simulink model "nonlinear_model"  (R2017b)
settings: Solver=VariableStepAuto  StartTime=0.0  StopTime=5  RelTol=1e-3
values from neighbouring files (symbols this model uses):
  altitude = input('Enter the altitude for the simulation (ft)  :  ')    [FindF16Dynamics.m]    (also in run_me.m = input(' altitude ( 0 ~ 40000 ft ) : '); trim_F16.m = alt)
  control_trim = u0    [find_trim.m]
  state_trim = steady_state( state )    [find_trim.m]
  velocity = input('Enter the velocity for the simulation (ft/s):  ')    [FindF16Dynamics.m]    (also in run_me.m = input(' true velocity ( 350 ~ 1000 ft/sec ) : '); trim_F16.m = vel)
libraries: simulink x7
settings Model: Creator=monster  LastModifiedBy=monster

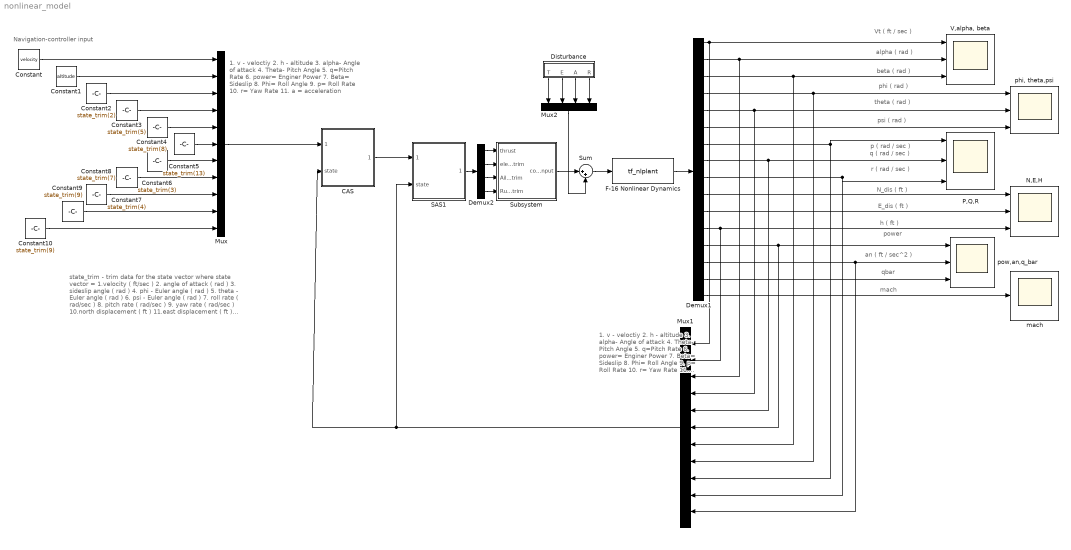
== system nonlinear_model ==
  note: state_trim   - trim data for the state vector where
      |       state vector =
      | 1.velocity             ( ft/sec )
      | 2. angle of attack      ( rad )
      |  3. sideslip angle       ( rad )
      | 4. phi   - Euler angle  ( rad )
      | 5. theta - Euler angle  ( rad )
      |    6. psi   - Euler angle  ( rad )
      |   7. roll rate            ( rad/sec )
      | 8. pitch rate           ( rad/sec )
      |  9. yaw rate             ( rad/sec )
      | 10.north displacement   ( ft )
      | 11.east displacement    ( ft )
      | 12.altitude             ( ft )
      | 13.power  ( percent, 0 <= pow <= 100 )
  note: phi ( rad )
  note: theta ( rad )
  note: h ( ft )
  note: E_dis ( ft )
  note: power
  note: an ( ft / sec^2 )
  note: mach
  note: Vt ( ft / sec )
  note: p ( rad / sec )
  note: r ( rad / sec )
  note: q ( rad / sec )
  note: N_dis ( ft )
  note: qbar
  note: alpha ( rad )
  note: beta ( rad )
  note: psi ( rad )
  note: 1. v - veloctiy
      |
      | 2. h - altitude
      |
      | 3. alpha- Angle of attack
      |
      | 4. Theta- Pitch Angle
      |
      | 5. q=Pitch Rate
      |
      | 6. power= Enginer Power
      |
      | 7. Beta= Sideslip
      |
      | 8. Phi= Roll Angle
      |
      | 9. p= Roll Rate
      |
      | 10. r= Yaw Rate
      |
      | 11. a = acceleration
  note: 1. v - veloctiy
      |
      | 2. h - altitude
      |
      | 3. alpha- Angle of attack
      |
      | 4. Theta- Pitch Angle
      |
      | 5. q=Pitch Rate
      |
      | 6. power= Enginer Power
      |
      | 7. Beta= Sideslip
      |
      | 8. Phi= Roll Angle
      |
      | 9. p= Roll Rate
      |
      | 10. r= Yaw Rate
      |
      | 11. a= acceleration
  note: Navigation-controller input
  " Disturbance" : Subsystem
  CAS : Subsystem
  Constant : Constant  Value=velocity
  Constant1 : Constant  Value=altitude
  Constant10 : Constant  Value=state_trim(9)
  Constant2 : Constant  Value=state_trim(2)
  Constant3 : Constant  Value=state_trim(5)
  Constant4 : Constant  Value=state_trim(8)
  Constant5 : Constant  Value=state_trim(13)
  Constant6 : Constant  Value=state_trim(3)
  Constant7 : Constant  Value=state_trim(4)
  Constant8 : Constant  Value=state_trim(7)
  Constant9 : Constant  Value=state_trim(9)
  Demux1 : Demux  Outputs=16
  Demux2 : Demux
  F-16 Nonlinear Dynamics : S-Function  FunctionName=tf_nlplant  Parameters="state_trim,  xcg"  SFunctionDeploymentMode=off  EnableBusSupport=off
  Mux : Mux  Inputs=11
  Mux1 : Mux  Inputs=11
  Mux2 : Mux
  N,E,H : Scope  NumInputPorts=3
  P,Q,R : Scope  NumInputPorts=3
  SAS1 : Subsystem
  Subsystem : Subsystem
  Sum : Sum  Inputs=|++
  "V,alpha, beta" : Scope  NumInputPorts=3
  mach : Scope
  "phi, theta,psi" : Scope  NumInputPorts=3
  pow,an,q_bar : Scope  NumInputPorts=3
  wires:
  Demux1/11 -> N,E,H/2
  Demux1/12 -> N,E,H/3, Mux1/2
  Demux1/1 -> Mux1/1, "V,alpha, beta"/1
  Demux1/15 -> pow,an,q_bar/3
  Demux1/2 -> "V,alpha, beta"/2, Mux1/3
  Demux1/4 -> Mux1/8, "phi, theta,psi"/1
  Demux1/9 -> Mux1/10, P,Q,R/3
  Demux1/8 -> Mux1/5, P,Q,R/2
  Demux1/10 -> N,E,H/1
  Demux1/5 -> Mux1/4, "phi, theta,psi"/2
  Demux1/3 -> Mux1/7, "V,alpha, beta"/3
  Demux1/7 -> Mux1/9, P,Q,R/1
  Demux1/6 -> "phi, theta,psi"/3
  Demux1/16 -> mach/1
  Demux1/13 -> Mux1/6, pow,an,q_bar/1
  " Disturbance"/3(A) -> Mux2/3
  " Disturbance"/2(E) -> Mux2/2
  Constant/1 -> Mux/1
  Constant9/1 -> Mux/10
  Constant6/1 -> Mux/7
  Constant2/1 -> Mux/3
  Constant1/1 -> Mux/2
  Constant4/1 -> Mux/5
  " Disturbance"/1(T) -> Mux2/1
  Constant7/1 -> Mux/8
  Constant8/1 -> Mux/9
  Constant3/1 -> Mux/4
  Demux2/4 -> Subsystem/4(Rudder_trim)
  Demux2/1 -> Subsystem/1(thrust)
  Demux2/2 -> Subsystem/2(elevator_trim)
  Subsystem/1(control_input) -> Sum/1
  Mux/1 -> CAS/1(reference)
  Constant10/1 -> Mux/11
  Constant5/1 -> Mux/6
  Sum/1 -> F-16 Nonlinear Dynamics/1
  Demux2/3 -> Subsystem/3(Aileron_trim)
  Mux2/1 -> Sum/2
  " Disturbance"/4(R) -> Mux2/4
  SAS1/1(control_input) -> Demux2/1
  F-16 Nonlinear Dynamics/1 -> Demux1/1
  Demux1/14 -> Mux1/11, pow,an,q_bar/2
  Mux1/1 -> SAS1/2(state), CAS/2(state)
  CAS/1(control_input) -> SAS1/1(reference)

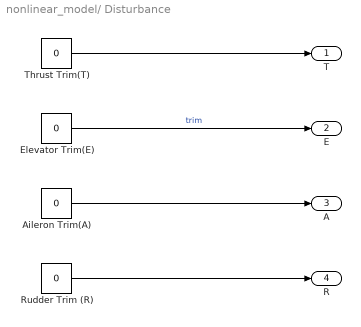
== system nonlinear_model/ Disturbance ==
  "Aileron Trim(A) " : Constant  Value=0
  "Elevator Trim(E) " : Constant  Value=0  VectorParams1D=off
  Rudder Trim (R) : Constant  Value=0
  "Thrust Trim(T) " : Constant  Value=0
  T : Outport
  E : Outport  Port=2
  A : Outport  Port=3
  R : Outport  Port=4
  wires:
  "Aileron Trim(A) "/1 -> A/1
  "Elevator Trim(E) "/1 -> E/1  "trim"
  "Thrust Trim(T) "/1 -> T/1
  Rudder Trim (R)/1 -> R/1

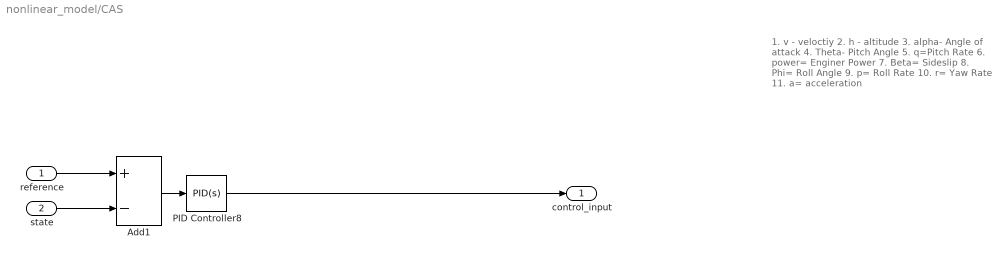
== system nonlinear_model/CAS ==
  note: 1. v - veloctiy
      |
      | 2. h - altitude
      |
      | 3. alpha- Angle of attack
      |
      | 4. Theta- Pitch Angle
      |
      | 5. q=Pitch Rate
      |
      | 6. power= Enginer Power
      |
      | 7. Beta= Sideslip
      |
      | 8. Phi= Roll Angle
      |
      | 9. p= Roll Rate
      |
      | 10. r= Yaw Rate
      |
      | 11. a= acceleration
  reference : Inport
  state : Inport  Port=2
  Add1 : Sum  Inputs=+-
  PID Controller8 : simulink/Continuous/PID Controller  Controller=PID  TimeDomain=Continuous-time  SampleTime=-1  IntegratorMethod=Forward Euler  FilterMethod=Forward Euler  Form=Parallel  UseFilter=on  ControllerParametersSource=internal  P=-49327.5398646116  I=-459229.123376859  D=-1288.80480278299  N=1181.77739704053  InitialConditionSource=internal  InitialConditionForIntegrator=0  InitialConditionForFilter=0  ExternalReset=none  LimitOutput=off  UpperSaturationLimit=inf  LowerSaturationLimit=-inf  LinearizeAsGain=on  AntiWindupMode=none  Kb=1  TrackingMode=off  Kt=1  PParamMin=[]  PParamMax=[]  IParamMin=[]  IParamMax=[]  DParamMin=[]  DParamMax=[]  NParamMin=[]  NParamMax=[]  KbParamMin=[]  KbParamMax=[]  KtParamMin=[]  KtParamMax=[]  POutMin=[]  POutMax=[]  IOutMin=[]  IOutMax=[]  DOutMin=[]  DOutMax=[]  NOutMin=[]  NOutMax=[]  KbOutMin=[]  KbOutMax=[]  KtOutMin=[]  KtOutMax=[]  IntegratorOutMin=[]  IntegratorOutMax=[]  FilterOutMin=[]  FilterOutMax=[]  SumOutMin=[]  SumOutMax=[]  SumI1OutMin=[]  SumI1OutMax=[]  SumI2OutMin=[]  SumI2OutMax=[]  SumI3OutMin=[]  SumI3OutMax=[]  SumDOutMin=[]  SumDOutMax=[]  SaturationOutMin=[]  SaturationOutMax=[]  IntegratorContinuousStateAttributes=''  IntegratorStateMustResolveToSignalObject=off  IntegratorRTWStateStorageClass=Auto  FilterContinuousStateAttributes=''  FilterStateMustResolveToSignalObject=off  FilterRTWStateStorageClass=Auto  DifferentiatorICPrevScaledInput=0  DifferentiatorOutMin=[]  DifferentiatorOutMax=[]  InitialConditionSetting=State (most efficient)  FilterDiffOutCoefMin=[]  FilterDiffOutCoefMax=[]  SumDenOutMin=[]  SumDenOutMax=[]  SumNumOutMin=[]  SumNumOutMax=[]  ReciprocalOutMin=[]  ReciprocalOutMax=[]  DivideOutMin=[]  DivideOutMax=[]  TunerSelectOption=Transfer Function Based (PID Tuner App)
  control_input : Outport
  wires:
  PID Controller8/1 -> control_input/1
  Add1/1 -> PID Controller8/1
  reference/1 -> Add1/1
  state/1 -> Add1/2

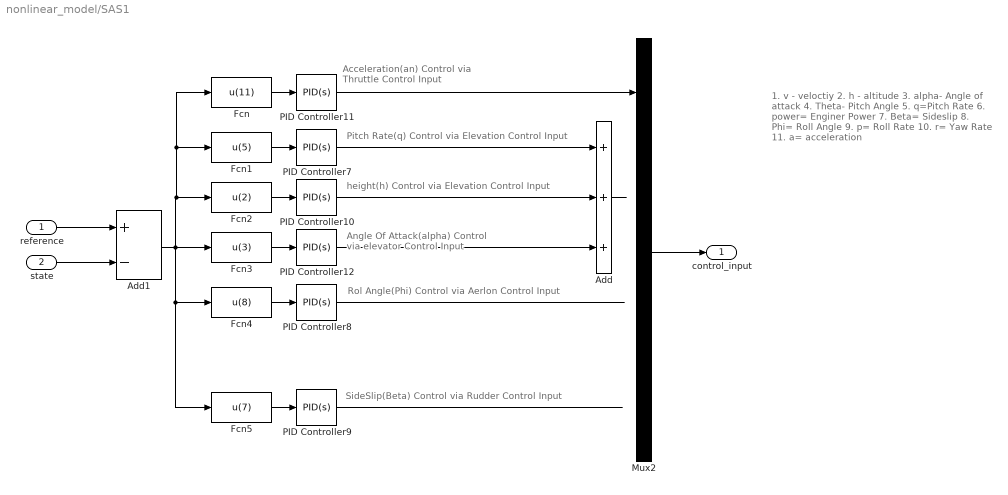
== system nonlinear_model/SAS1 ==
  note: Rol Angle(Phi) Control via Aerlon Control Input
  note: height(h) Control via Elevation Control Input
  note: Pitch Rate(q) Control via Elevation Control Input
  note: Acceleration(an) Control via Thruttle Control Input
  note: Angle Of Attack(alpha) Control via elevator Control Input
  note: SideSlip(Beta) Control via Rudder Control Input
  note: 1. v - veloctiy
      |
      | 2. h - altitude
      |
      | 3. alpha- Angle of attack
      |
      | 4. Theta- Pitch Angle
      |
      | 5. q=Pitch Rate
      |
      | 6. power= Enginer Power
      |
      | 7. Beta= Sideslip
      |
      | 8. Phi= Roll Angle
      |
      | 9. p= Roll Rate
      |
      | 10. r= Yaw Rate
      |
      | 11. a= acceleration
  reference : Inport
  state : Inport  Port=2
  Add : Sum  Inputs=+++
  Add1 : Sum  Inputs=+-
  Fcn : Fcn  Expr=u(11)
  Fcn1 : Fcn  Expr=u(5)
  Fcn2 : Fcn  Expr=u(2)
  Fcn3 : Fcn  Expr=u(3)
  Fcn4 : Fcn  Expr=u(8)
  Fcn5 : Fcn  Expr=u(7)
  Mux2 : Mux
  PID Controller10 : simulink/Continuous/PID Controller  Controller=PID  TimeDomain=Continuous-time  SampleTime=-1  IntegratorMethod=Forward Euler  FilterMethod=Forward Euler  Form=Parallel  UseFilter=on  ControllerParametersSource=internal  P=24508600.1259152  I=4501969741.89748  D=28958.3047379278  N=690409.793644926  InitialConditionSource=internal  InitialConditionForIntegrator=0  InitialConditionForFilter=0  ExternalReset=none  LimitOutput=off  UpperSaturationLimit=inf  LowerSaturationLimit=-inf  LinearizeAsGain=on  AntiWindupMode=none  Kb=1  TrackingMode=off  Kt=1  PParamMin=[]  PParamMax=[]  IParamMin=[]  IParamMax=[]  DParamMin=[]  DParamMax=[]  NParamMin=[]  NParamMax=[]  KbParamMin=[]  KbParamMax=[]  KtParamMin=[]  KtParamMax=[]  POutMin=[]  POutMax=[]  IOutMin=[]  IOutMax=[]  DOutMin=[]  DOutMax=[]  NOutMin=[]  NOutMax=[]  KbOutMin=[]  KbOutMax=[]  KtOutMin=[]  KtOutMax=[]  IntegratorOutMin=[]  IntegratorOutMax=[]  FilterOutMin=[]  FilterOutMax=[]  SumOutMin=[]  SumOutMax=[]  SumI1OutMin=[]  SumI1OutMax=[]  SumI2OutMin=[]  SumI2OutMax=[]  SumI3OutMin=[]  SumI3OutMax=[]  SumDOutMin=[]  SumDOutMax=[]  SaturationOutMin=[]  SaturationOutMax=[]  IntegratorContinuousStateAttributes=''  IntegratorStateMustResolveToSignalObject=off  IntegratorRTWStateStorageClass=Auto  FilterContinuousStateAttributes=''  FilterStateMustResolveToSignalObject=off  FilterRTWStateStorageClass=Auto  DifferentiatorICPrevScaledInput=0  DifferentiatorOutMin=[]  DifferentiatorOutMax=[]  InitialConditionSetting=State (most efficient)  FilterDiffOutCoefMin=[]  FilterDiffOutCoefMax=[]  SumDenOutMin=[]  SumDenOutMax=[]  SumNumOutMin=[]  SumNumOutMax=[]  ReciprocalOutMin=[]  ReciprocalOutMax=[]  DivideOutMin=[]  DivideOutMax=[]  TunerSelectOption=Transfer Function Based (PID Tuner App)
  PID Controller11 : simulink/Continuous/PID Controller  Controller=PID  TimeDomain=Continuous-time  SampleTime=-1  IntegratorMethod=Forward Euler  FilterMethod=Forward Euler  Form=Parallel  UseFilter=on  ControllerParametersSource=internal  P=13329483.1324469  I=392847306.175743  D=98980.5300334758  N=109037.560099343  InitialConditionSource=internal  InitialConditionForIntegrator=0  InitialConditionForFilter=0  ExternalReset=none  LimitOutput=off  UpperSaturationLimit=inf  LowerSaturationLimit=-inf  LinearizeAsGain=on  AntiWindupMode=none  Kb=1  TrackingMode=off  Kt=1  PParamMin=[]  PParamMax=[]  IParamMin=[]  IParamMax=[]  DParamMin=[]  DParamMax=[]  NParamMin=[]  NParamMax=[]  KbParamMin=[]  KbParamMax=[]  KtParamMin=[]  KtParamMax=[]  POutMin=[]  POutMax=[]  IOutMin=[]  IOutMax=[]  DOutMin=[]  DOutMax=[]  NOutMin=[]  NOutMax=[]  KbOutMin=[]  KbOutMax=[]  KtOutMin=[]  KtOutMax=[]  IntegratorOutMin=[]  IntegratorOutMax=[]  FilterOutMin=[]  FilterOutMax=[]  SumOutMin=[]  SumOutMax=[]  SumI1OutMin=[]  SumI1OutMax=[]  SumI2OutMin=[]  SumI2OutMax=[]  SumI3OutMin=[]  SumI3OutMax=[]  SumDOutMin=[]  SumDOutMax=[]  SaturationOutMin=[]  SaturationOutMax=[]  IntegratorContinuousStateAttributes=''  IntegratorStateMustResolveToSignalObject=off  IntegratorRTWStateStorageClass=Auto  FilterContinuousStateAttributes=''  FilterStateMustResolveToSignalObject=off  FilterRTWStateStorageClass=Auto  DifferentiatorICPrevScaledInput=0  DifferentiatorOutMin=[]  DifferentiatorOutMax=[]  InitialConditionSetting=State (most efficient)  FilterDiffOutCoefMin=[]  FilterDiffOutCoefMax=[]  SumDenOutMin=[]  SumDenOutMax=[]  SumNumOutMin=[]  SumNumOutMax=[]  ReciprocalOutMin=[]  ReciprocalOutMax=[]  DivideOutMin=[]  DivideOutMax=[]  TunerSelectOption=Transfer Function Based (PID Tuner App)
  PID Controller12 : simulink/Continuous/PID Controller  Controller=PID  TimeDomain=Continuous-time  SampleTime=-1  IntegratorMethod=Forward Euler  FilterMethod=Forward Euler  Form=Parallel  UseFilter=on  ControllerParametersSource=internal  P=-170.14183467408  I=-465.695324804371  D=-13.6839697818054  N=105.697856042613  InitialConditionSource=internal  InitialConditionForIntegrator=0  InitialConditionForFilter=0  ExternalReset=none  LimitOutput=off  UpperSaturationLimit=inf  LowerSaturationLimit=-inf  LinearizeAsGain=on  AntiWindupMode=none  Kb=1  TrackingMode=off  Kt=1  PParamMin=[]  PParamMax=[]  IParamMin=[]  IParamMax=[]  DParamMin=[]  DParamMax=[]  NParamMin=[]  NParamMax=[]  KbParamMin=[]  KbParamMax=[]  KtParamMin=[]  KtParamMax=[]  POutMin=[]  POutMax=[]  IOutMin=[]  IOutMax=[]  DOutMin=[]  DOutMax=[]  NOutMin=[]  NOutMax=[]  KbOutMin=[]  KbOutMax=[]  KtOutMin=[]  KtOutMax=[]  IntegratorOutMin=[]  IntegratorOutMax=[]  FilterOutMin=[]  FilterOutMax=[]  SumOutMin=[]  SumOutMax=[]  SumI1OutMin=[]  SumI1OutMax=[]  SumI2OutMin=[]  SumI2OutMax=[]  SumI3OutMin=[]  SumI3OutMax=[]  SumDOutMin=[]  SumDOutMax=[]  SaturationOutMin=[]  SaturationOutMax=[]  IntegratorContinuousStateAttributes=''  IntegratorStateMustResolveToSignalObject=off  IntegratorRTWStateStorageClass=Auto  FilterContinuousStateAttributes=''  FilterStateMustResolveToSignalObject=off  FilterRTWStateStorageClass=Auto  DifferentiatorICPrevScaledInput=0  DifferentiatorOutMin=[]  DifferentiatorOutMax=[]  InitialConditionSetting=State (most efficient)  FilterDiffOutCoefMin=[]  FilterDiffOutCoefMax=[]  SumDenOutMin=[]  SumDenOutMax=[]  SumNumOutMin=[]  SumNumOutMax=[]  ReciprocalOutMin=[]  ReciprocalOutMax=[]  DivideOutMin=[]  DivideOutMax=[]  TunerSelectOption=Transfer Function Based (PID Tuner App)
  PID Controller7 : simulink/Continuous/PID Controller  Controller=PID  TimeDomain=Continuous-time  SampleTime=-1  IntegratorMethod=Forward Euler  FilterMethod=Forward Euler  Form=Parallel  UseFilter=on  ControllerParametersSource=internal  P=-2409.99420452658  I=-41171.6281036838  D=-4.63151383685818  N=352.425457454863  InitialConditionSource=internal  InitialConditionForIntegrator=0  InitialConditionForFilter=0  ExternalReset=none  LimitOutput=off  UpperSaturationLimit=inf  LowerSaturationLimit=-inf  LinearizeAsGain=on  AntiWindupMode=none  Kb=1  TrackingMode=off  Kt=1  PParamMin=[]  PParamMax=[]  IParamMin=[]  IParamMax=[]  DParamMin=[]  DParamMax=[]  NParamMin=[]  NParamMax=[]  KbParamMin=[]  KbParamMax=[]  KtParamMin=[]  KtParamMax=[]  POutMin=[]  POutMax=[]  IOutMin=[]  IOutMax=[]  DOutMin=[]  DOutMax=[]  NOutMin=[]  NOutMax=[]  KbOutMin=[]  KbOutMax=[]  KtOutMin=[]  KtOutMax=[]  IntegratorOutMin=[]  IntegratorOutMax=[]  FilterOutMin=[]  FilterOutMax=[]  SumOutMin=[]  SumOutMax=[]  SumI1OutMin=[]  SumI1OutMax=[]  SumI2OutMin=[]  SumI2OutMax=[]  SumI3OutMin=[]  SumI3OutMax=[]  SumDOutMin=[]  SumDOutMax=[]  SaturationOutMin=[]  SaturationOutMax=[]  IntegratorContinuousStateAttributes=''  IntegratorStateMustResolveToSignalObject=off  IntegratorRTWStateStorageClass=Auto  FilterContinuousStateAttributes=''  FilterStateMustResolveToSignalObject=off  FilterRTWStateStorageClass=Auto  DifferentiatorICPrevScaledInput=0  DifferentiatorOutMin=[]  DifferentiatorOutMax=[]  InitialConditionSetting=State (most efficient)  FilterDiffOutCoefMin=[]  FilterDiffOutCoefMax=[]  SumDenOutMin=[]  SumDenOutMax=[]  SumNumOutMin=[]  SumNumOutMax=[]  ReciprocalOutMin=[]  ReciprocalOutMax=[]  DivideOutMin=[]  DivideOutMax=[]  TunerSelectOption=Transfer Function Based (PID Tuner App)
  PID Controller8 : simulink/Continuous/PID Controller  Controller=PID  TimeDomain=Continuous-time  SampleTime=-1  IntegratorMethod=Forward Euler  FilterMethod=Forward Euler  Form=Parallel  UseFilter=on  ControllerParametersSource=internal  P=-49327.5398646116  I=-459229.123376859  D=-1288.80480278299  N=1181.77739704053  InitialConditionSource=internal  InitialConditionForIntegrator=0  InitialConditionForFilter=0  ExternalReset=none  LimitOutput=off  UpperSaturationLimit=inf  LowerSaturationLimit=-inf  LinearizeAsGain=on  AntiWindupMode=none  Kb=1  TrackingMode=off  Kt=1  PParamMin=[]  PParamMax=[]  IParamMin=[]  IParamMax=[]  DParamMin=[]  DParamMax=[]  NParamMin=[]  NParamMax=[]  KbParamMin=[]  KbParamMax=[]  KtParamMin=[]  KtParamMax=[]  POutMin=[]  POutMax=[]  IOutMin=[]  IOutMax=[]  DOutMin=[]  DOutMax=[]  NOutMin=[]  NOutMax=[]  KbOutMin=[]  KbOutMax=[]  KtOutMin=[]  KtOutMax=[]  IntegratorOutMin=[]  IntegratorOutMax=[]  FilterOutMin=[]  FilterOutMax=[]  SumOutMin=[]  SumOutMax=[]  SumI1OutMin=[]  SumI1OutMax=[]  SumI2OutMin=[]  SumI2OutMax=[]  SumI3OutMin=[]  SumI3OutMax=[]  SumDOutMin=[]  SumDOutMax=[]  SaturationOutMin=[]  SaturationOutMax=[]  IntegratorContinuousStateAttributes=''  IntegratorStateMustResolveToSignalObject=off  IntegratorRTWStateStorageClass=Auto  FilterContinuousStateAttributes=''  FilterStateMustResolveToSignalObject=off  FilterRTWStateStorageClass=Auto  DifferentiatorICPrevScaledInput=0  DifferentiatorOutMin=[]  DifferentiatorOutMax=[]  InitialConditionSetting=State (most efficient)  FilterDiffOutCoefMin=[]  FilterDiffOutCoefMax=[]  SumDenOutMin=[]  SumDenOutMax=[]  SumNumOutMin=[]  SumNumOutMax=[]  ReciprocalOutMin=[]  ReciprocalOutMax=[]  DivideOutMin=[]  DivideOutMax=[]  TunerSelectOption=Transfer Function Based (PID Tuner App)
  PID Controller9 : simulink/Continuous/PID Controller  Controller=PID  TimeDomain=Continuous-time  SampleTime=-1  IntegratorMethod=Forward Euler  FilterMethod=Forward Euler  Form=Parallel  UseFilter=on  ControllerParametersSource=internal  P=908.491475757153  I=143.160579860217  D=1280.97081759687  N=3086.89831654681  InitialConditionSource=internal  InitialConditionForIntegrator=0  InitialConditionForFilter=0  ExternalReset=none  LimitOutput=off  UpperSaturationLimit=inf  LowerSaturationLimit=-inf  LinearizeAsGain=on  AntiWindupMode=none  Kb=1  TrackingMode=off  Kt=1  PParamMin=[]  PParamMax=[]  IParamMin=[]  IParamMax=[]  DParamMin=[]  DParamMax=[]  NParamMin=[]  NParamMax=[]  KbParamMin=[]  KbParamMax=[]  KtParamMin=[]  KtParamMax=[]  POutMin=[]  POutMax=[]  IOutMin=[]  IOutMax=[]  DOutMin=[]  DOutMax=[]  NOutMin=[]  NOutMax=[]  KbOutMin=[]  KbOutMax=[]  KtOutMin=[]  KtOutMax=[]  IntegratorOutMin=[]  IntegratorOutMax=[]  FilterOutMin=[]  FilterOutMax=[]  SumOutMin=[]  SumOutMax=[]  SumI1OutMin=[]  SumI1OutMax=[]  SumI2OutMin=[]  SumI2OutMax=[]  SumI3OutMin=[]  SumI3OutMax=[]  SumDOutMin=[]  SumDOutMax=[]  SaturationOutMin=[]  SaturationOutMax=[]  IntegratorContinuousStateAttributes=''  IntegratorStateMustResolveToSignalObject=off  IntegratorRTWStateStorageClass=Auto  FilterContinuousStateAttributes=''  FilterStateMustResolveToSignalObject=off  FilterRTWStateStorageClass=Auto  DifferentiatorICPrevScaledInput=0  DifferentiatorOutMin=[]  DifferentiatorOutMax=[]  InitialConditionSetting=State (most efficient)  FilterDiffOutCoefMin=[]  FilterDiffOutCoefMax=[]  SumDenOutMin=[]  SumDenOutMax=[]  SumNumOutMin=[]  SumNumOutMax=[]  ReciprocalOutMin=[]  ReciprocalOutMax=[]  DivideOutMin=[]  DivideOutMax=[]  TunerSelectOption=Transfer Function Based (PID Tuner App)
  control_input : Outport
  wires:
  Mux2/1 -> control_input/1
  PID Controller11/1 -> Mux2/1
  Fcn5/1 -> PID Controller9/1
  Fcn3/1 -> PID Controller12/1
  PID Controller7/1 -> Add/1
  Fcn2/1 -> PID Controller10/1
  Fcn1/1 -> PID Controller7/1
  PID Controller8/1 -> ?
  Fcn4/1 -> PID Controller8/1
  Fcn/1 -> PID Controller11/1
  PID Controller10/1 -> Add/2
  Add/1 -> ?
  PID Controller12/1 -> Add/3
  PID Controller9/1 -> ?
  reference/1 -> Add1/1
  state/1 -> Add1/2
  Add1/1 -> Fcn2/1, Fcn1/1, Fcn/1, Fcn5/1, Fcn4/1, Fcn3/1

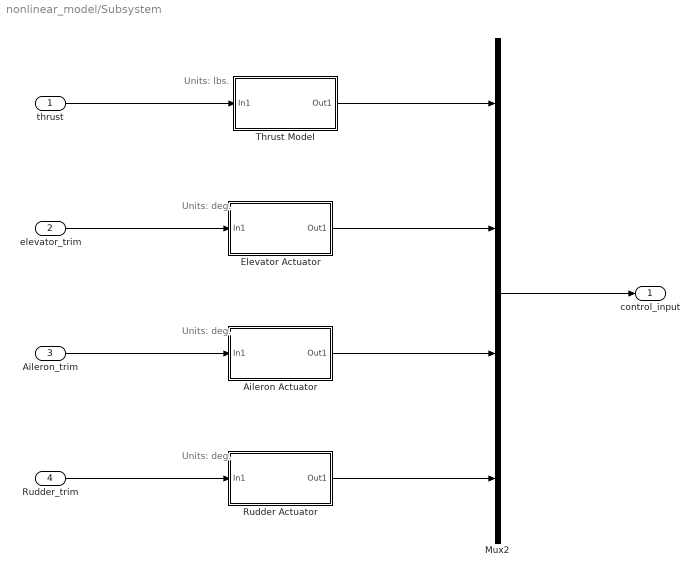
== system nonlinear_model/Subsystem ==
  note: Units: deg.
  note: Units: deg.
  note: Units: lbs.
  note: Units: deg.
  thrust : Inport
  elevator_trim : Inport  Port=2
  Aileron_trim : Inport  Port=3
  Rudder_trim : Inport  Port=4
  Aileron Actuator : Subsystem  AncestorBlock=F16_Actuator_Library/Aileron Actuator
  Elevator Actuator : Subsystem  AncestorBlock=F16_Actuator_Library/Elevator Actuator
  Mux2 : Mux
  Rudder Actuator : Subsystem  AncestorBlock=F16_Actuator_Library/Rudder Actuator
  Thrust Model : Subsystem  AncestorBlock=F16_Actuator_Library/Thrust Model
  control_input : Outport
  wires:
  thrust/1 -> Thrust Model/1(In1)
  Aileron Actuator/1(Out1) -> Mux2/3
  Rudder_trim/1 -> Rudder Actuator/1(In1)
  Elevator Actuator/1(Out1) -> Mux2/2
  Rudder Actuator/1(Out1) -> Mux2/4
  elevator_trim/1 -> Elevator Actuator/1(In1)
  Aileron_trim/1 -> Aileron Actuator/1(In1)
  Thrust Model/1(Out1) -> Mux2/1
  Mux2/1 -> control_input/1

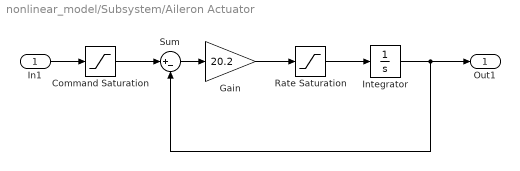
== system nonlinear_model/Subsystem/Aileron Actuator ==
  In1 : Inport
  Command Saturation : Saturate  UpperLimit=21.5  LowerLimit=-21.5
  Gain : Gain  Gain=20.2  SaturateOnIntegerOverflow=on  OutDataTypeStr=Inherit: Same as input  ParamDataTypeStr=Inherit: Same as input
  "Integrator " : Integrator  InitialCondition=control_trim(2)  UpperSaturationLimit=21.5  LowerSaturationLimit=-21.5
  Rate Saturation : Saturate  UpperLimit=80  LowerLimit=-80
  Sum : Sum  Inputs=|+-  SaturateOnIntegerOverflow=on  InputSameDT=on  OutDataTypeStr=Inherit: Same as first input
  Out1 : Outport
  wires:
  "Integrator "/1 -> Sum/2, Out1/1
  Rate Saturation/1 -> "Integrator "/1
  Gain/1 -> Rate Saturation/1
  Sum/1 -> Gain/1
  Command Saturation/1 -> Sum/1
  In1/1 -> Command Saturation/1

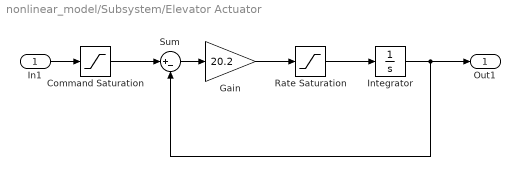
== system nonlinear_model/Subsystem/Elevator Actuator ==
  In1 : Inport
  Command Saturation : Saturate  UpperLimit=25  LowerLimit=-25
  Gain : Gain  Gain=20.2  SaturateOnIntegerOverflow=on  OutDataTypeStr=Inherit: Same as input  ParamDataTypeStr=Inherit: Same as input
  "Integrator " : Integrator  InitialCondition=control_trim(2)  UpperSaturationLimit=25  LowerSaturationLimit=-25
  Rate Saturation : Saturate  UpperLimit=60  LowerLimit=-60
  Sum : Sum  Inputs=|+-  SaturateOnIntegerOverflow=on  InputSameDT=on  OutDataTypeStr=Inherit: Same as first input
  Out1 : Outport
  wires:
  "Integrator "/1 -> Sum/2, Out1/1
  Rate Saturation/1 -> "Integrator "/1
  Gain/1 -> Rate Saturation/1
  Sum/1 -> Gain/1
  Command Saturation/1 -> Sum/1
  In1/1 -> Command Saturation/1

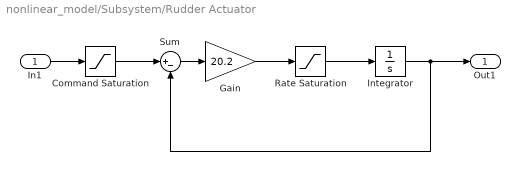
== system nonlinear_model/Subsystem/Rudder Actuator ==
  In1 : Inport
  Command Saturation : Saturate  UpperLimit=30  LowerLimit=-30
  Gain : Gain  Gain=20.2  SaturateOnIntegerOverflow=on  OutDataTypeStr=Inherit: Same as input  ParamDataTypeStr=Inherit: Same as input
  "Integrator " : Integrator  InitialCondition=control_trim(2)  UpperSaturationLimit=30  LowerSaturationLimit=-30
  Rate Saturation : Saturate  UpperLimit=120  LowerLimit=-120
  Sum : Sum  Inputs=|+-  SaturateOnIntegerOverflow=on  InputSameDT=on  OutDataTypeStr=Inherit: Same as first input
  Out1 : Outport
  wires:
  "Integrator "/1 -> Sum/2, Out1/1
  Rate Saturation/1 -> "Integrator "/1
  Gain/1 -> Rate Saturation/1
  Sum/1 -> Gain/1
  Command Saturation/1 -> Sum/1
  In1/1 -> Command Saturation/1

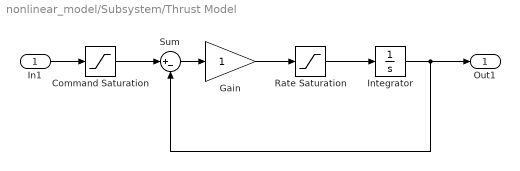
== system nonlinear_model/Subsystem/Thrust Model ==
  In1 : Inport
  Command Saturation : Saturate  UpperLimit=19000  LowerLimit=1000
  Gain : Gain  SaturateOnIntegerOverflow=on  OutDataTypeStr=Inherit: Same as input  ParamDataTypeStr=Inherit: Same as input
  "Integrator " : Integrator  InitialCondition=control_trim(1)  UpperSaturationLimit=30  LowerSaturationLimit=-30
  Rate Saturation : Saturate  UpperLimit=19000  LowerLimit=1000
  Sum : Sum  Inputs=|+-  SaturateOnIntegerOverflow=on  InputSameDT=on  OutDataTypeStr=Inherit: Same as first input
  Out1 : Outport
  wires:
  "Integrator "/1 -> Sum/2, Out1/1
  Rate Saturation/1 -> "Integrator "/1
  Gain/1 -> Rate Saturation/1
  Sum/1 -> Gain/1
  Command Saturation/1 -> Sum/1
  In1/1 -> Command Saturation/1
